simulink model "Grp43_assign2_2"  (R2023a)
settings: Solver=VariableStepAuto  StartTime=0.0  StopTime=7  RelTol=1e-3
values from neighbouring files (symbols this model uses):
  a0 = double(sol.a0)    [Grp43_part2_code.m]    (also in e01 2.m = double(S.a0); grp43_asgn2_2.m = double(S.a0))
  a1 = double(sol.a1)    [Grp43_part2_code.m]    (also in e01 2.m = double(S.a1); grp43_asgn2_2.m = double(S.a1))
  g = 9.8    [Grp43_Code.m]    (also in Grp43_part2_code.m = 9.81; e01 2.m; grp43_asgn2_2.m)
  l = 0.36    [Grp43_Code.m]    (also in Grp43_part2_code.m; e01 2.m; grp43_asgn2_2.m)
  m = 0.26    [Grp43_Code.m]    (also in Grp43_part2_code.m; e01 2.m; grp43_asgn2_2.m)
  M = 2.4    [Grp43_Code.m]    (also in Grp43_part2_code.m; e01 2.m; grp43_asgn2_2.m)
  p0 = double(sol.p0)    [Grp43_part2_code.m]    (also in e01 2.m = double(S.p0); grp43_asgn2_2.m = double(S.p0))
  p1 = double(sol.p1)    [Grp43_part2_code.m]    (also in e01 2.m = double(S.p1); grp43_asgn2_2.m = double(S.p1))
  q0 = double(sol.q0)    [Grp43_part2_code.m]    (also in e01 2.m = double(S.q0); grp43_asgn2_2.m = double(S.q0))
settings Model: Creator=jitbi  LastModifiedBy=Anirvan Krishna

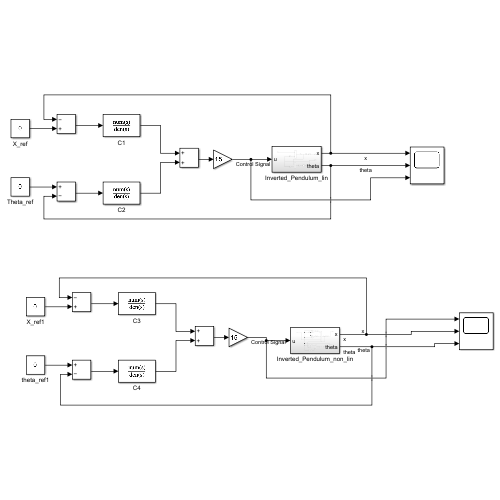
[thumbnail: Simulink's stored preview of the top-level diagram]
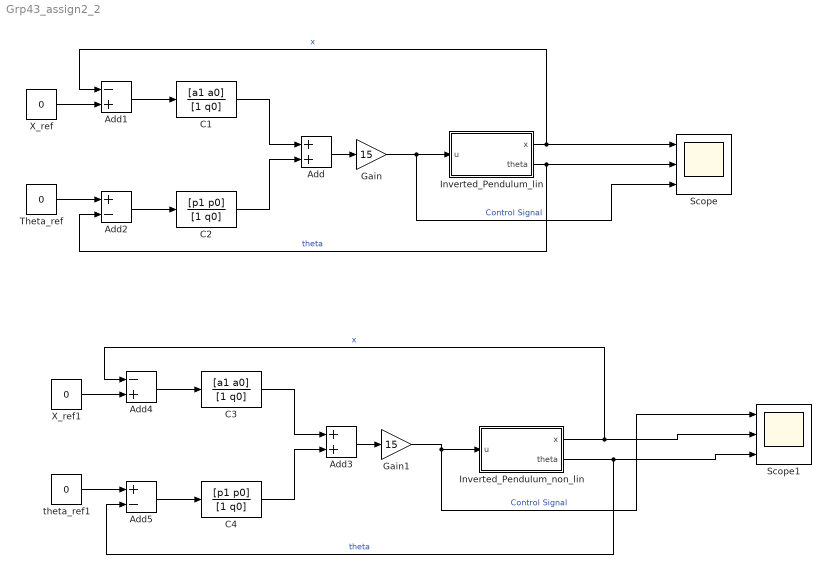
== system Grp43_assign2_2 ==
  Add : Sum
  Add1 : Sum  Inputs=-+
  Add2 : Sum  Inputs=+-
  Add3 : Sum
  Add4 : Sum  Inputs=-+
  Add5 : Sum  Inputs=+-
  C1 : TransferFcn  Numerator=[a1 a0]  Denominator=[1 q0]
  C2 : TransferFcn  Numerator=[p1 p0]  Denominator=[1 q0]
  C3 : TransferFcn  Numerator=[a1 a0]  Denominator=[1 q0]
  C4 : TransferFcn  Numerator=[p1 p0]  Denominator=[1 q0]
  Gain : Gain  Gain=15
  Gain1 : Gain  Gain=15
  Inverted_Pendulum_lin : Subsystem
  Inverted_Pendulum_non_lin : Subsystem
  Scope : Scope  NumInputPorts=3
  Scope1 : Scope  NumInputPorts=3
  Theta_ref : Constant  Value=0
  X_ref : Constant  Value=0
  X_ref1 : Constant  Value=0
  theta_ref1 : Constant  Value=0
  wires:
  C1/1 -> Add/1
  C2/1 -> Add/2
  X_ref/1 -> Add1/2
  Add1/1 -> C1/1
  Theta_ref/1 -> Add2/1
  Add2/1 -> C2/1
  Add/1 -> Gain/1
  Inverted_Pendulum_lin/1(x) -> Scope/1, Add1/1  "x"
  Inverted_Pendulum_lin/2(theta) -> Add2/2, Scope/2  "theta"
  Gain/1 -> Scope/3, Inverted_Pendulum_lin/1(u)  "Control Signal"
  Gain1/1 -> Scope1/1, Inverted_Pendulum_non_lin/1(u)  "Control Signal"
  Inverted_Pendulum_non_lin/2(theta) -> Add5/2, Scope1/3  "theta"
  theta_ref1/1 -> Add5/1
  Inverted_Pendulum_non_lin/1(x) -> Add4/1, Scope1/2  "x"
  C4/1 -> Add3/2
  Add4/1 -> C3/1
  Add3/1 -> Gain1/1
  X_ref1/1 -> Add4/2
  Add5/1 -> C4/1
  C3/1 -> Add3/1

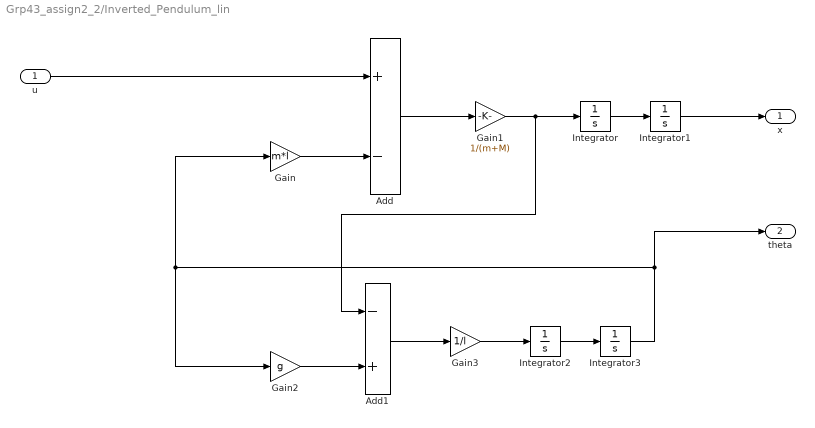
== system Grp43_assign2_2/Inverted_Pendulum_lin ==
  u : Inport
  Add : Sum  Inputs=+-
  Add1 : Sum  Inputs=-+
  Gain : Gain  Gain=m*l
  Gain1 : Gain  Gain=1/(m+M)
  Gain2 : Gain  Gain=g
  Gain3 : Gain  Gain=1/l
  Integrator : Integrator
  Integrator1 : Integrator
  Integrator2 : Integrator
  Integrator3 : Integrator  InitialCondition=1e-10
  x : Outport
  theta : Outport  Port=2
  wires:
  u/1 -> Add/1
  Gain/1 -> Add/2
  Integrator3/1 -> theta/1, Gain/1, Gain2/1
  Add/1 -> Gain1/1
  Integrator/1 -> Integrator1/1
  Gain1/1 -> Add1/1, Integrator/1
  Integrator1/1 -> x/1
  Gain2/1 -> Add1/2
  Add1/1 -> Gain3/1
  Integrator2/1 -> Integrator3/1
  Gain3/1 -> Integrator2/1

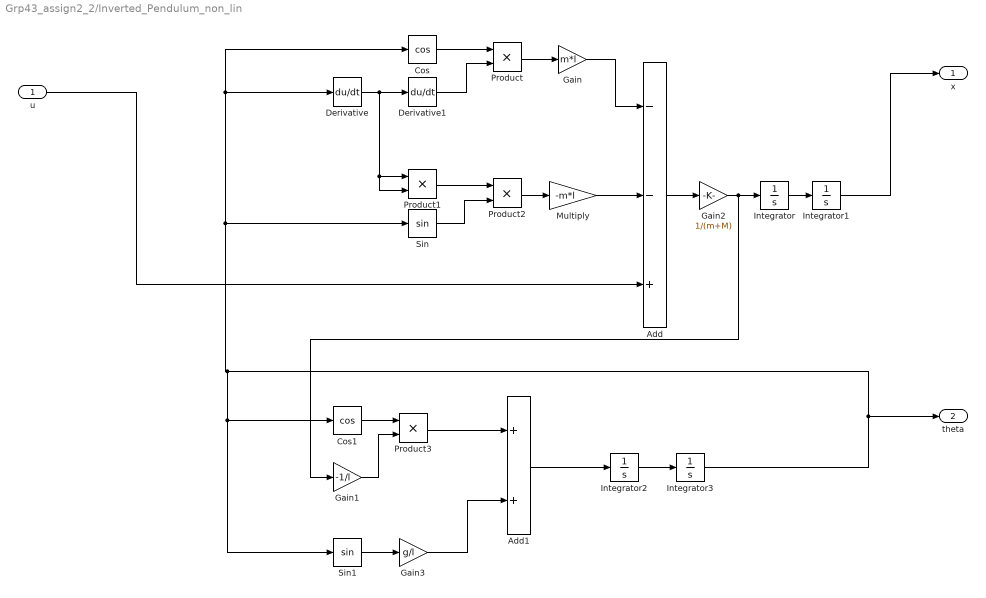
== system Grp43_assign2_2/Inverted_Pendulum_non_lin ==
  u : Inport
  Add : Sum  Inputs=--+
  Add1 : Sum
  Cos : Trigonometry  Operator=cos
  Cos1 : Trigonometry  Operator=cos
  Derivative : Derivative
  Derivative1 : Derivative
  Gain : Gain  Gain=m*l
  Gain1 : Gain  Gain=-1/l
  Gain2 : Gain  Gain=1/(m+M)
  Gain3 : Gain  Gain=g/l
  Integrator : Integrator
  Integrator1 : Integrator
  Integrator2 : Integrator
  Integrator3 : Integrator  InitialCondition=1e-10
  Multiply : Gain  Gain=-m*l
  Product{,1..3} (4 alike) : Product
  Sin : Trigonometry
  Sin1 : Trigonometry
  x : Outport
  theta : Outport  Port=2
  wires:
  Product2/1 -> Multiply/1
  Integrator3/1 -> Cos1/1, Sin1/1, Cos/1, Derivative/1, Sin/1, theta/1
  Add/1 -> Gain2/1
  Cos/1 -> Product/1
  Derivative/1 -> Product1/1, Product1/2, Derivative1/1
  u/1 -> Add/3
  Derivative1/1 -> Product/2
  Product/1 -> Gain/1
  Multiply/1 -> Add/2
  Integrator/1 -> Integrator1/1
  Gain2/1 -> Gain1/1, Integrator/1
  Product1/1 -> Product2/1
  Sin/1 -> Product2/2
  Gain/1 -> Add/1
  Integrator1/1 -> x/1
  Cos1/1 -> Product3/1
  Gain1/1 -> Product3/2
  Sin1/1 -> Gain3/1
  Product3/1 -> Add1/1
  Gain3/1 -> Add1/2
  Add1/1 -> Integrator2/1
  Integrator2/1 -> Integrator3/1
